simulink model "simulacao_485"  (R2021b)
settings: Solver=VariableStepAuto  StartTime=0.0  StopTime=0.0016  RelTol=1e-3
libraries: ee_lib x1
settings Model: Creator=harmonia  LastModifiedBy=harmonia

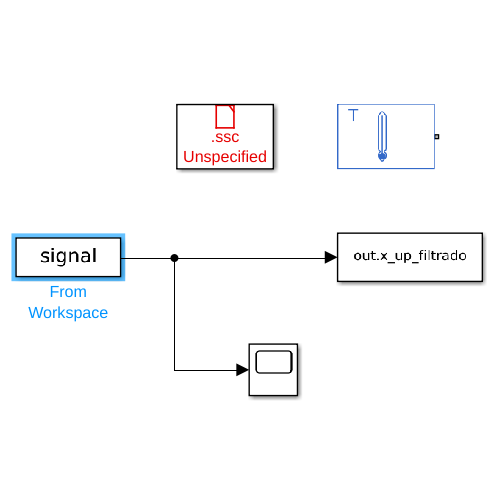
[thumbnail: Simulink's stored preview of the top-level diagram]
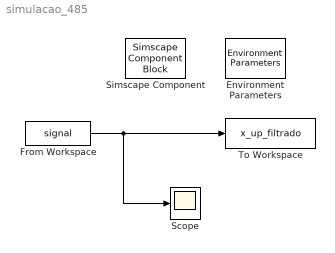
== system simulacao_485 ==
  Environment Parameters : ee_lib/Utilities/Environment Parameters  Temperature=300.15 K  GMIN=1e-12 1/Ohm
      settings: SourceProductBaseCode=PS  InternalSimscapePortConfiguration="{\"Bottom\":[],\"Left\":[],\"Right\":[{\"id\":\"E\",\"label\":\"\",\"type\":\"foundation.electrical.electrical\"}],\"Top\":[]}"
  From Workspace : FromWorkspace  VariableName=signal  OutDataTypeStr=double  Interpolate=off  ZeroCross=off  OutputAfterFinalValue=Holding final value
  Scope : Scope
  Simscape Component : SimscapeComponentBlock
      settings: CopyFcn=simscape.engine.sli.internal.componentblockcallback(gcbh,'COPY')  PreCopyFcn=simscape.engine.sli.internal.componentblockcallback(gcbh,'PRECOPY')  PreDeleteFcn=simscape.engine.sli.internal.componentblockcallback(gcbh,'PREDELETE')
      mask Display: color('red');plot([0 1 1 0 0],[0 0 1 1 0]);plot([0.7,1],[1,0.7]);plot(-2,-1.75);plot(3, 1);disp('\n.ssc\nUnspecified')
  To Workspace : ToWorkspace  VariableName=x_up_filtrado  SampleTime=t(2)-t(1)
      settings: Save2DSignal=2-D array (concatenate along first dimension)
  wires:
  From Workspace/1 -> To Workspace/1, Scope/1
